simulink model "simulacija_fitriranja_signala"  (R2018a)
settings: Solver=VariableStepAuto  StartTime=0.0  StopTime=1.0  RelTol=1e-3
values from neighbouring files (symbols this model uses):
  K = 45    [z2.m]
settings Model: Creator=djoco  LastModifiedBy=djoco

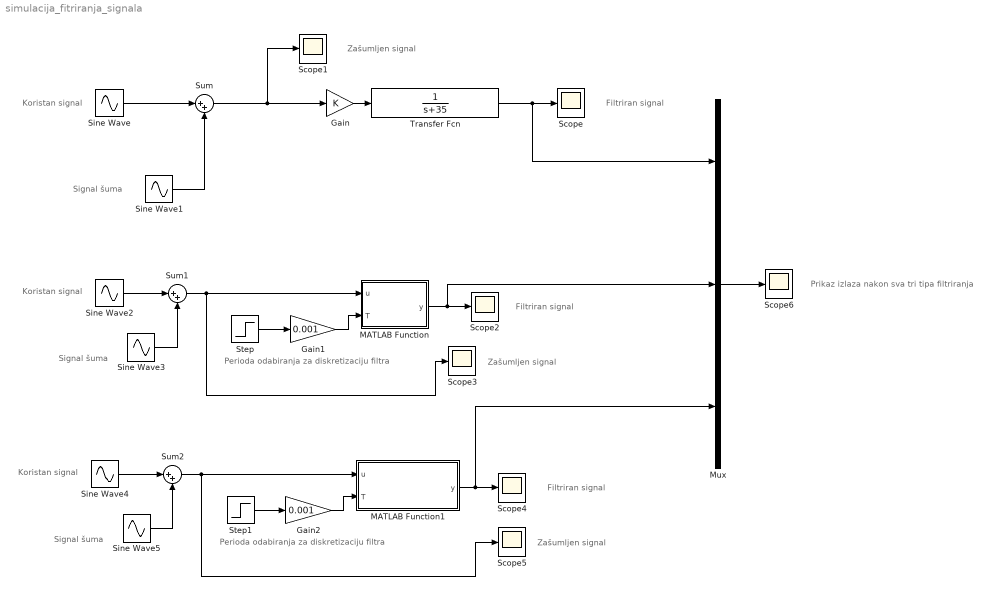
== system simulacija_fitriranja_signala ==
  note: Prikaz izlaza nakon sva tri tipa filtriranja
  note: Filtriran signal
  note: Signal šuma
  note: Perioda odabiranja za diskretizaciju filtra
  note: Zašumljen signal
  note: Koristan signal
  note: Signal šuma
  note: Koristan signal
  note: Zašumljen signal
  note: Filtriran signal
  note: Perioda odabiranja za diskretizaciju filtra
  note: Zašumljen signal
  note: Signal šuma
  note: Filtriran signal
  note: Koristan signal
  Gain : Gain  Gain=K
  Gain1 : Gain  Gain=0.001
  Gain2 : Gain  Gain=0.001
  MATLAB Function : MATLAB Function  TreatAsAtomicUnit=on
  MATLAB Function1 : MATLAB Function  TreatAsAtomicUnit=on
  Mux : Mux  Inputs=3
  Scope{,1..6} (7 alike) : Scope
  Sine Wave : Sin  Frequency=30  SampleTime=0
  Sine Wave1 : Sin  Frequency=1500  SampleTime=0
  Sine Wave2 : Sin  Frequency=30  SampleTime=0
  Sine Wave3 : Sin  Frequency=1500  SampleTime=0
  Sine Wave4 : Sin  Frequency=30  SampleTime=0
  Sine Wave5 : Sin  Frequency=1500  SampleTime=0
  Step : Step  Time=0  Before=1  SampleTime=0
  Step1 : Step  Time=0  Before=1  SampleTime=0
  Sum : Sum  Inputs=|++
  Sum1 : Sum  Inputs=|++
  Sum2 : Sum  Inputs=|++
  Transfer Fcn : TransferFcn  Denominator=[1 35]
  wires:
  Sum/1 -> Gain/1, Scope1/1
  Sine Wave/1 -> Sum/1
  Sine Wave1/1 -> Sum/2
  Transfer Fcn/1 -> Mux/1, Scope/1
  Gain/1 -> Transfer Fcn/1
  Sine Wave3/1 -> Sum1/2
  Sum1/1 -> Scope3/1, MATLAB Function/1(u)
  Gain1/1 -> MATLAB Function/2(T)
  MATLAB Function/1(y) -> Mux/2, Scope2/1
  Sine Wave2/1 -> Sum1/1
  Step/1 -> Gain1/1
  Step1/1 -> Gain2/1
  Sum2/1 -> Scope5/1, MATLAB Function1/1(u)
  Gain2/1 -> MATLAB Function1/2(T)
  Sine Wave5/1 -> Sum2/2
  MATLAB Function1/1(y) -> Mux/3, Scope4/1
  Sine Wave4/1 -> Sum2/1
  Mux/1 -> Scope6/1

== matlab function simulacija_fitriranja_signala/MATLAB Function1 ==
  settings: updateMethod=DISCRETE
  data: u input; y output; T input
function y = step_inv_filtar(u, T)


persistent yp up

if isempty(yp)
    yp = 0;
end
if isempty(up)
    up = 0;
end


y = (45*(1 - exp(-35*T))/35)*up + exp(-35*T)*yp;

yp = y;
up = u;

== matlab function simulacija_fitriranja_signala/MATLAB Function ==
  settings: updateMethod=DISCRETE
  data: u input; y output; T input
function y = ojler_filtar(u, T)


persistent yp

if isempty(yp)
    yp = 0;
end


y = (45*T/(35*T+1))*u + (1/(35*T+1))*yp;

yp = y;
